simulink model "ClosedLoop_Test"  (R2023b)
settings: Solver=VariableStepAuto  StartTime=0.0  StopTime=10.0  RelTol=1e-3
libraries: cstblocks x7
settings Model: Creator=randolf  LastModifiedBy=randolf

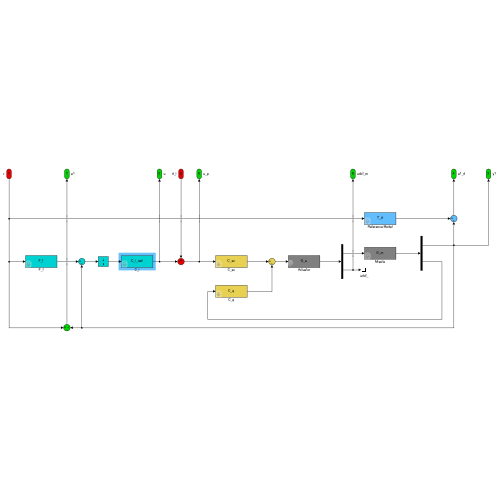
[thumbnail: Simulink's stored preview of the top-level diagram]
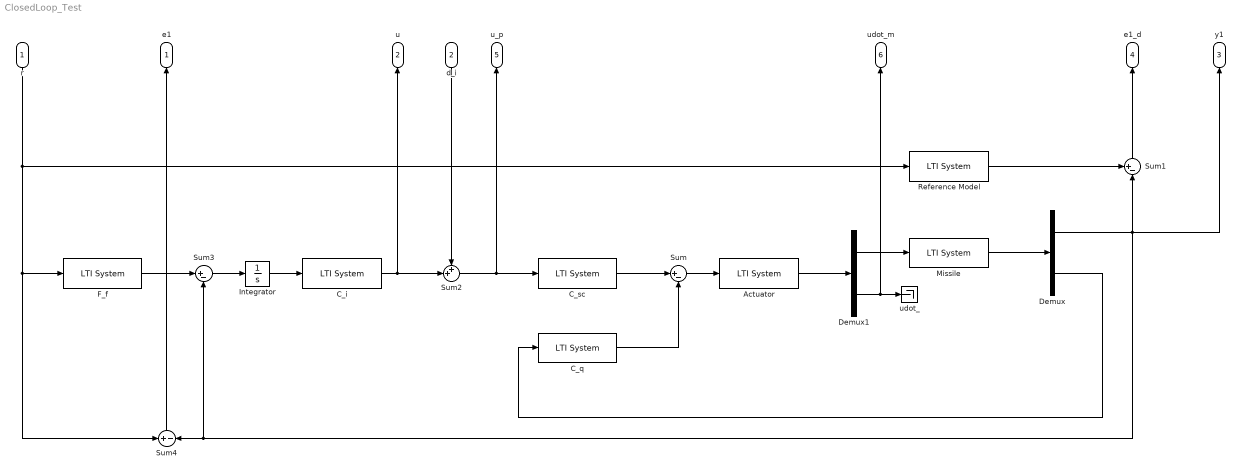
== system ClosedLoop_Test ==
  r : Inport
  d_i : Inport  Port=2
  Actuator : cstblocks/LTI System  sys=G_a  IC=[]  PadeOrder=0
  C_i : cstblocks/LTI System  sys=C_i  IC=[]  PadeOrder=0
  C_q : cstblocks/LTI System  sys=C_q  IC=[]  PadeOrder=0
  C_sc : cstblocks/LTI System  sys=C_sc  IC=[]  PadeOrder=0
  Demux : Demux  Outputs=2
  Demux1 : Demux  Outputs=2
  F_f : cstblocks/LTI System  sys=F_f  IC=[]  PadeOrder=0
  Integrator : Integrator
  Missile : cstblocks/LTI System  sys=G_m  IC=[]  PadeOrder=0
  Reference Model : cstblocks/LTI System  sys=T_d  IC=[]  PadeOrder=0
  Sum : Sum  Inputs=|+-
  Sum1 : Sum  Inputs=+-|
  Sum2 : Sum  Inputs=++|
  Sum3 : Sum  Inputs=|+-
  Sum4 : Sum  Inputs=+|-
  udot_ : Terminator
  e1 : Outport
  u : Outport  Port=2
  y1 : Outport  Port=3
  e1_d : Outport  Port=4
  u_p : Outport  Port=5
  udot_m : Outport  Port=6
  wires:
  C_q/1 -> Sum/2
  Sum/1 -> Actuator/1
  Missile/1 -> Demux/1
  Demux1/1 -> Missile/1
  C_sc/1 -> Sum/1
  Actuator/1 -> Demux1/1
  Demux/2 -> C_q/1
  Demux1/2 -> udot_m/1, udot_/1
  Sum2/1 -> u_p/1, C_sc/1
  C_i/1 -> u/1, Sum2/2
  Integrator/1 -> C_i/1
  Sum3/1 -> Integrator/1
  F_f/1 -> Sum3/1
  Reference Model/1 -> Sum1/1
  Demux/1 -> y1/1, Sum3/2, Sum4/2, Sum1/2
  r/1 -> Reference Model/1, Sum4/1, F_f/1
  d_i/1 -> Sum2/1
  Sum4/1 -> e1/1
  Sum1/1 -> e1_d/1
